simulink model "simulatore"  (R2024a)
settings: Solver=VariableStepAuto  StartTime=0.0  StopTime=0  RelTol=1e-3
values from neighbouring files (symbols this model uses):
  alpharad = (alpha*pi)/180    [cl_alpha.m]
  cd0 = 0.01    [cambio_performance.m]    (also in simulazione_trimmaggio.m; verfica_validazione.m)
  Cl = ext_nl_CLalfa_XLS(:,2)'    [cl_alpha.m]
  deltaT_conv = (T/(n_engine*Tsl) )*(rho0/rhoz)^nt    [simulazione_trimmaggio.m]
  e = 0.9    [simulazione_trimmaggio.m]
  g = 9.8066    [cambio_performance.m]    (also in simulazione_trimmaggio.m; verfica_validazione.m)
  height_des = height_trim+(1000*0.3048)    (= 1219.2)    [simulazione_trimmaggio.m]
  height_trim = h_ft * 0.3048    [cambio_performance.m]    (also in simulazione_trimmaggio.m = 914.4; verfica_validazione.m)
  lambda = -0.0065    [cambio_performance.m]    (also in simulazione_trimmaggio.m; verfica_validazione.m)
  lambdaD = (wing_span^2) / wing_area    (= 8.57002616279)    [cambio_performance.m]    (also in simulazione_trimmaggio.m; verfica_validazione.m)
  MFC = (2144+2122)*0.4535    (= 1934.631)    [simulazione_trimmaggio.m]
  MTOM = 9163    [cambio_performance.m]    (also in simulazione_trimmaggio.m; verfica_validazione.m)
  nt = 1.4236    [simulazione_trimmaggio.m]
  phiT = (8*pi)/180    (= 0.13962634016)    [cambio_performance.m]    (also in simulazione_trimmaggio.m = 0; verfica_validazione.m = 0)
  R = 287.05    [cambio_performance.m]    (also in simulazione_trimmaggio.m; verfica_validazione.m)
  rho0 = 1.225    [cambio_performance.m]    (also in simulazione_trimmaggio.m; verfica_validazione.m)
  SFC = 0.44*0.45/(0.45*9.81/1000*3600)    (= 0.0124589421226)    [simulazione_trimmaggio.m]
  T0 = 288.15    [cambio_performance.m]    (also in simulazione_trimmaggio.m; verfica_validazione.m)
  thetaT = alphaT+gammaT    (= 0.0349065850399)    [simulazione_trimmaggio.m]
  Tsl = 18.32*(10^3)    (= 18320)    [simulazione_trimmaggio.m]
  v = Mach * Vs    [cambio_performance.m]    (also in simulazione_trimmaggio.m = Mach*Vs; verfica_validazione.m)
  wing_area = 34.4    [cambio_performance.m]    (also in simulazione_trimmaggio.m; verfica_validazione.m)
undefined symbols (not defined in the file or in its folder): magnitude
settings Model: Creator=lisys  LastModifiedBy=Simone

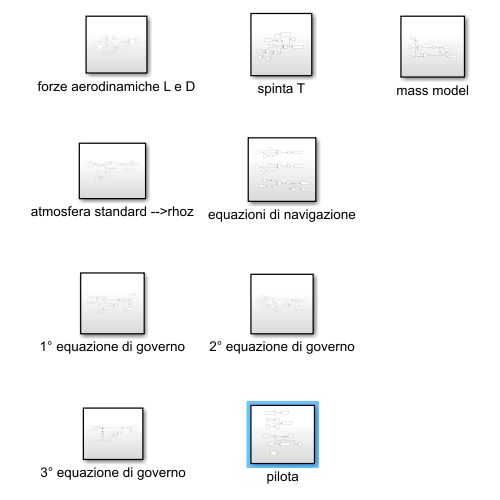
[thumbnail: Simulink's stored preview of the top-level diagram]
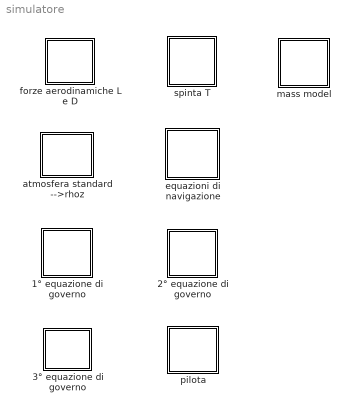
== system simulatore ==
  1° equazione di governo : Subsystem
  2° equazione di governo : Subsystem
  3° equazione di governo : Subsystem
  atmosfera standard -->rhoz : Subsystem
  equazioni di navigazione : Subsystem
  forze aerodinamiche L e D : Subsystem
  mass model : Subsystem
  pilota : Subsystem
  spinta T : Subsystem

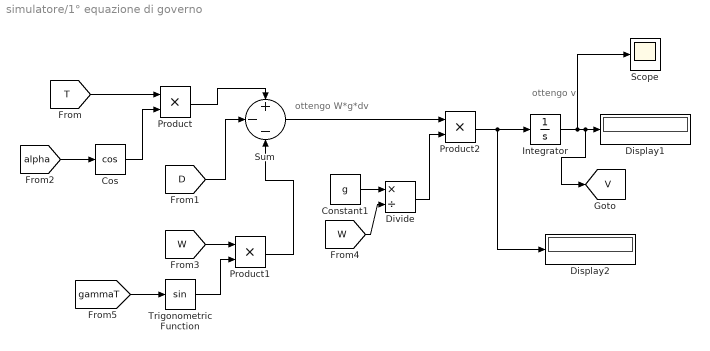
== system simulatore/1° equazione di governo ==
  note: ottengo v
  note: ottengo W*g*dv
  Constant1 : Constant  Value=g
  Cos : Trigonometry  Operator=cos
  Display1 : Display
  Display2 : Display
  Divide : Product  Inputs=*/
  Integrator : Integrator  InitialCondition=v
  Product : Product
  Product1 : Product
  Product2 : Product
  Scope : Scope
  Sum : Sum  Inputs=+--
  Trigonometric Function : Trigonometry
  tag scope: V=global
  wires:
  Integrator/1 -> Scope/1, [V], Display1/1
  [alpha] -> Cos/1
  Trigonometric Function/1 -> Product1/2
  [D] -> Sum/2
  Sum/1 -> Product2/1
  Cos/1 -> Product/2
  Constant1/1 -> Divide/1
  [W] -> Product1/1
  [T] -> Product/1
  Product/1 -> Sum/1
  Divide/1 -> Product2/2
  Product1/1 -> Sum/3
  [W] -> Divide/2
  [gammaT] -> Trigonometric Function/1
  Product2/1 -> Display2/1, Integrator/1

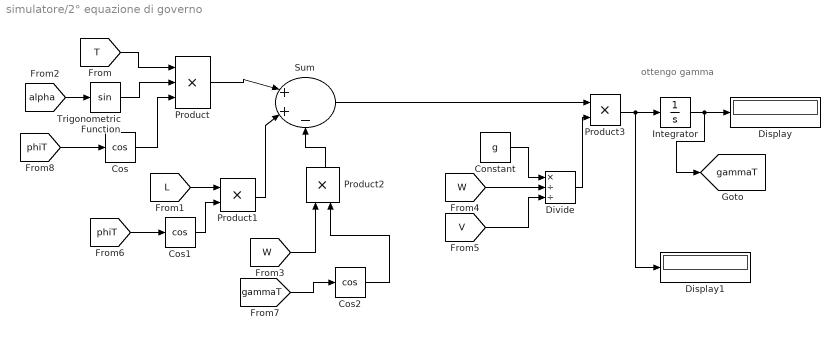
== system simulatore/2° equazione di governo ==
  note: ottengo gamma
  Constant : Constant  Value=g
  Cos : Trigonometry  Operator=cos
  Cos1 : Trigonometry  Operator=cos
  Cos2 : Trigonometry  Operator=cos
  Display : Display
  Display1 : Display
  Divide : Product  Inputs=*//
  Integrator : Integrator
  Product : Product  Inputs=3
  Product1 : Product
  Product2 : Product
  Product3 : Product
  Sum : Sum  Inputs=|++-
  Trigonometric Function : Trigonometry
  tag scope: gammaT=global
  wires:
  Product1/1 -> Sum/2
  [alpha] -> Trigonometric Function/1
  [L] -> Product1/1
  Sum/1 -> Product3/1
  Integrator/1 -> [gammaT], Display/1
  [W] -> Divide/2
  Product2/1 -> Sum/3
  Cos2/1 -> Product2/2
  Cos1/1 -> Product1/2
  Product/1 -> Sum/1
  Divide/1 -> Product3/2
  Cos/1 -> Product/3
  Trigonometric Function/1 -> Product/2
  [W] -> Product2/1
  Product3/1 -> Display1/1, Integrator/1
  [T] -> Product/1
  [phiT] -> Cos1/1
  [gammaT] -> Cos2/1
  [phiT] -> Cos/1
  Constant/1 -> Divide/1
  [V] -> Divide/3

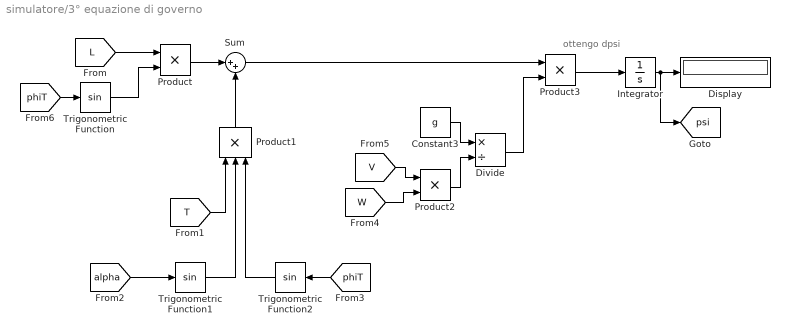
== system simulatore/3° equazione di governo ==
  note: ottengo dpsi
  Constant3 : Constant  Value=g
  Display : Display
  Divide : Product  Inputs=*/
  Integrator : Integrator
  Product : Product
  Product1 : Product  Inputs=3
  Product2 : Product
  Product3 : Product
  Sum : Sum  Inputs=|++
  Trigonometric Function : Trigonometry
  Trigonometric Function1 : Trigonometry
  Trigonometric Function2 : Trigonometry
  tag scope: psi=global
  wires:
  Sum/1 -> Product3/1
  Trigonometric Function/1 -> Product/2
  Product2/1 -> Divide/2
  [alpha] -> Trigonometric Function1/1
  [W] -> Product2/2
  Divide/1 -> Product3/2
  [T] -> Product1/1
  Product3/1 -> Integrator/1
  Trigonometric Function2/1 -> Product1/3
  Integrator/1 -> [psi], Display/1
  Trigonometric Function1/1 -> Product1/2
  Product1/1 -> Sum/2
  Product/1 -> Sum/1
  [L] -> Product/1
  Constant3/1 -> Divide/1
  [V] -> Product2/1
  [phiT] -> Trigonometric Function2/1
  [phiT] -> Trigonometric Function/1

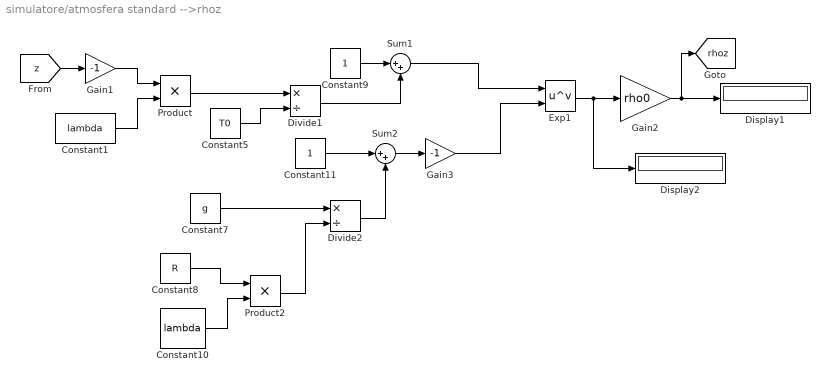
== system simulatore/atmosfera standard -->rhoz ==
  Constant1 : Constant  Value=lambda
  Constant10 : Constant  Value=lambda
  Constant11 : Constant
  Constant5 : Constant  Value=T0
  Constant7 : Constant  Value=g
  Constant8 : Constant  Value=R
  Constant9 : Constant
  Display1 : Display
  Display2 : Display
  Divide1 : Product  Inputs=*/
  Divide2 : Product  Inputs=*/
  Exp1 : Math  Operator=pow
  Gain1 : Gain  Gain=-1
  Gain2 : Gain  Gain=rho0
  Gain3 : Gain  Gain=-1
  Product : Product
  Product2 : Product
  Sum1 : Sum  Inputs=|++
  Sum2 : Sum  Inputs=|++
  tag scope: rhoz=global
  wires:
  Constant10/1 -> Product2/2
  Divide2/1 -> Sum2/2
  Constant5/1 -> Divide1/2
  Exp1/1 -> Display2/1, Gain2/1
  Constant7/1 -> Divide2/1
  Constant9/1 -> Sum1/1
  Constant8/1 -> Product2/1
  Divide1/1 -> Sum1/2
  Product2/1 -> Divide2/2
  Constant11/1 -> Sum2/1
  Sum1/1 -> Exp1/1
  Gain2/1 -> [rhoz], Display1/1
  [z] -> Gain1/1
  Sum2/1 -> Gain3/1
  Gain3/1 -> Exp1/2
  Gain1/1 -> Product/1
  Constant1/1 -> Product/2
  Product/1 -> Divide1/1

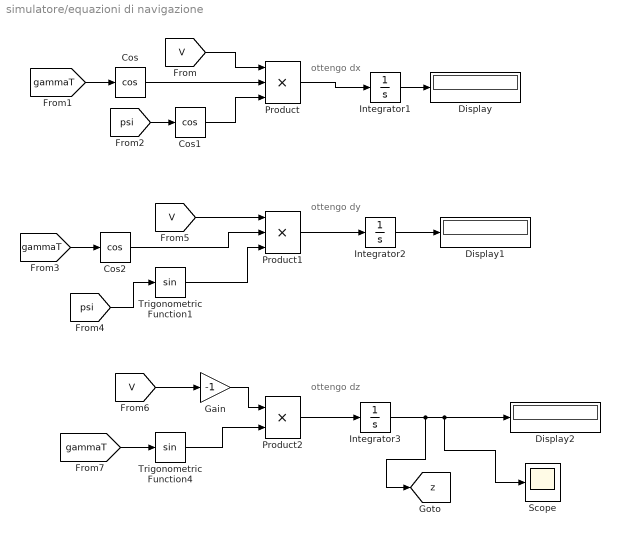
== system simulatore/equazioni di navigazione ==
  note: ottengo dx
  note: ottengo dy
  note: ottengo dz
  Cos : Trigonometry  Operator=cos
  Cos1 : Trigonometry  Operator=cos
  Cos2 : Trigonometry  Operator=cos
  Display : Display
  Display1 : Display
  Display2 : Display
  Gain : Gain  Gain=-1
  Integrator1 : Integrator
  Integrator2 : Integrator
  Integrator3 : Integrator  InitialCondition=-height_trim
  Product : Product  Inputs=3
  Product1 : Product  Inputs=3
  Product2 : Product
  Scope : Scope
  Trigonometric Function1 : Trigonometry
  Trigonometric Function4 : Trigonometry
  tag scope: z=global
  wires:
  Product1/1 -> Integrator2/1
  Product2/1 -> Integrator3/1
  Product/1 -> Integrator1/1
  Trigonometric Function4/1 -> Product2/2
  [V] -> Product/1
  Cos/1 -> Product/2
  Cos1/1 -> Product/3
  [gammaT] -> Cos/1
  [psi] -> Cos1/1
  Integrator1/1 -> Display/1
  Integrator2/1 -> Display1/1
  Cos2/1 -> Product1/2
  Trigonometric Function1/1 -> Product1/3
  [gammaT] -> Cos2/1
  [psi] -> Trigonometric Function1/1
  [V] -> Product1/1
  [V] -> Gain/1
  Gain/1 -> Product2/1
  [gammaT] -> Trigonometric Function4/1
  Integrator3/1 -> [z], Scope/1, Display2/1

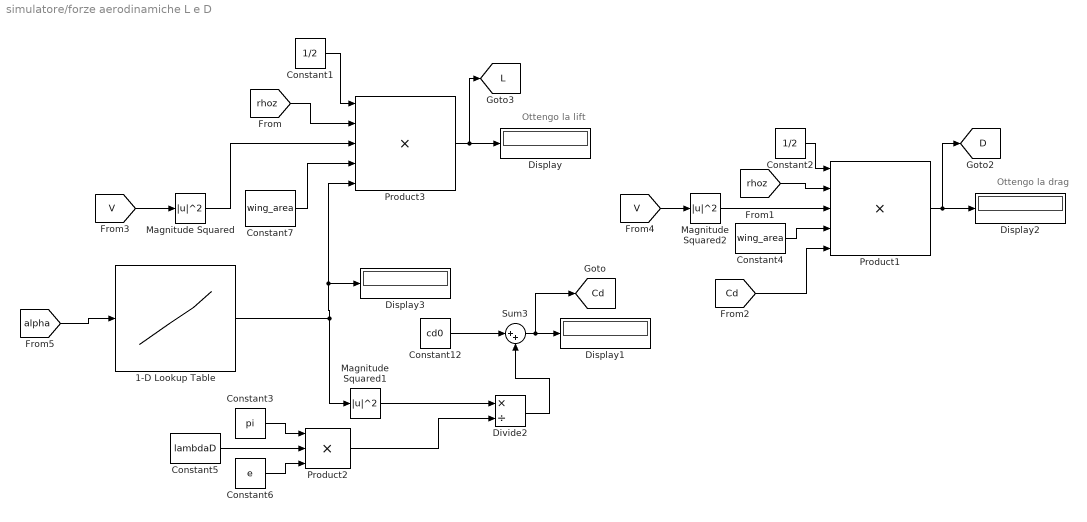
== system simulatore/forze aerodinamiche L e D ==
  note: Ottengo la lift
  note: Ottengo la drag
  1-D Lookup Table : Lookup_n-D  NumberOfTableDimensions=1  BreakpointsForDimension1=alpharad  Table=Cl  InternalRulePriority=Speed  RndMeth=Simplest
  Constant1 : Constant  Value=1/2
  Constant12 : Constant  Value=cd0
  Constant2 : Constant  Value=1/2
  Constant3 : Constant  Value=pi
  Constant4 : Constant  Value=wing_area
  Constant5 : Constant  Value=lambdaD
  Constant6 : Constant  Value=e
  Constant7 : Constant  Value=wing_area
  Display{,1..3} (4 alike) : Display
  Divide2 : Product  Inputs=*/
  Magnitude Squared : Math  Operator=magnitude^2
  Magnitude Squared1 : Math  Operator=magnitude^2
  Magnitude Squared2 : Math  Operator=magnitude^2
  Product1 : Product  Inputs=5
  Product2 : Product  Inputs=3
  Product3 : Product  Inputs=5
  Sum3 : Sum  Inputs=|++
  tag scope: Cd=global, D=global, L=global
  wires:
  Constant1/1 -> Product3/1
  Magnitude Squared1/1 -> Divide2/1
  Product3/1 -> [L], Display/1
  1-D Lookup Table/1 -> Magnitude Squared1/1, Display3/1, Product3/5
  Constant7/1 -> Product3/4
  Constant12/1 -> Sum3/1
  Magnitude Squared/1 -> Product3/3
  Divide2/1 -> Sum3/2
  Sum3/1 -> [Cd], Display1/1
  [rhoz] -> Product3/2
  [rhoz] -> Product1/2
  Magnitude Squared2/1 -> Product1/3
  Constant4/1 -> Product1/4
  Product1/1 -> [D], Display2/1
  Constant2/1 -> Product1/1
  [Cd] -> Product1/5
  [V] -> Magnitude Squared/1
  [V] -> Magnitude Squared2/1
  Constant3/1 -> Product2/1
  Constant5/1 -> Product2/2
  Constant6/1 -> Product2/3
  Product2/1 -> Divide2/2
  [alpha] -> 1-D Lookup Table/1

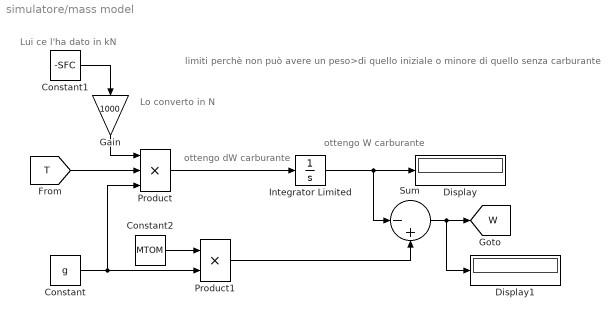
== system simulatore/mass model ==
  note: Lui ce l'ha dato in kN
  note: ottengo dW carburante
  note: limiti perchè non può avere un peso>di quello iniziale o minore di quello senza carburante
  note: ottengo W carburante
  note: Lo converto in N
  Constant : Constant  Value=g
  Constant1 : Constant  Value=-SFC
  Constant2 : Constant  Value=MTOM
  Display : Display
  Display1 : Display
  Gain : Gain  Gain=1000
  Integrator Limited : Integrator  LimitOutput=on  UpperSaturationLimit=MFC*g  LowerSaturationLimit=0
  Product : Product  Inputs=3
  Product1 : Product
  Sum : Sum  Inputs=|-+
  tag scope: W=global
  wires:
  Constant/1 -> Product/3, Product1/2
  Constant1/1 -> Gain/1
  Product/1 -> Integrator Limited/1
  Integrator Limited/1 -> Sum/1, Display/1
  Gain/1 -> Product/1
  Sum/1 -> Display1/1, [W]
  Constant2/1 -> Product1/1
  [T] -> Product/2
  Product1/1 -> Sum/2

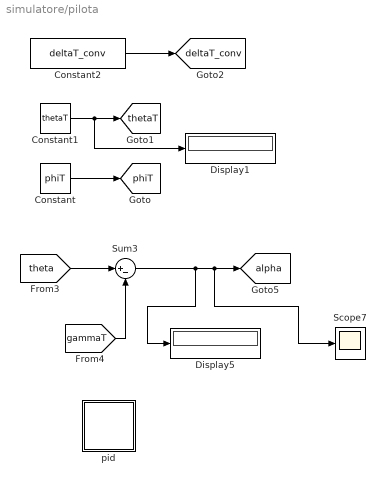
== system simulatore/pilota ==
  Constant : Constant  Value=phiT
  Constant1 : Constant  Value=thetaT
  Constant2 : Constant  Value=deltaT_conv
  Display1 : Display
  Display5 : Display
  Scope7 : Scope
  Sum3 : Sum  Inputs=|+-
  pid : Subsystem
  tag scope: alpha=global, deltaT_conv=global, phiT=global, thetaT=global
  wires:
  Constant/1 -> [phiT]
  Constant2/1 -> [deltaT_conv]
  Constant1/1 -> Display1/1, [thetaT]
  Sum3/1 -> Scope7/1, [alpha], Display5/1
  [theta] -> Sum3/1
  [gammaT] -> Sum3/2

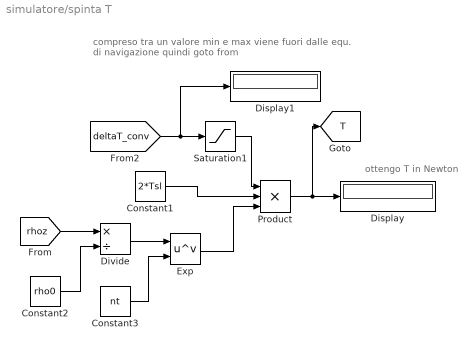
== system simulatore/spinta T ==
  note: compreso tra un valore min e max
      | viene fuori dalle equ. di navigazione quindi goto from
  note: ottengo T in Newton
  Constant1 : Constant  Value=2*Tsl
  Constant2 : Constant  Value=rho0
  Constant3 : Constant  Value=nt
  Display : Display
  Display1 : Display
  Divide : Product  Inputs=*/
  Exp : Math  Operator=pow
  Product : Product  Inputs=3
  Saturation1 : Saturate  UpperLimit=1  LowerLimit=0.015
  tag scope: T=global
  wires:
  Divide/1 -> Exp/1
  Constant2/1 -> Divide/2
  Product/1 -> [T], Display/1
  [rhoz] -> Divide/1
  Constant1/1 -> Product/2
  Constant3/1 -> Exp/2
  Exp/1 -> Product/3
  [deltaT_conv] -> Saturation1/1, Display1/1
  Saturation1/1 -> Product/1

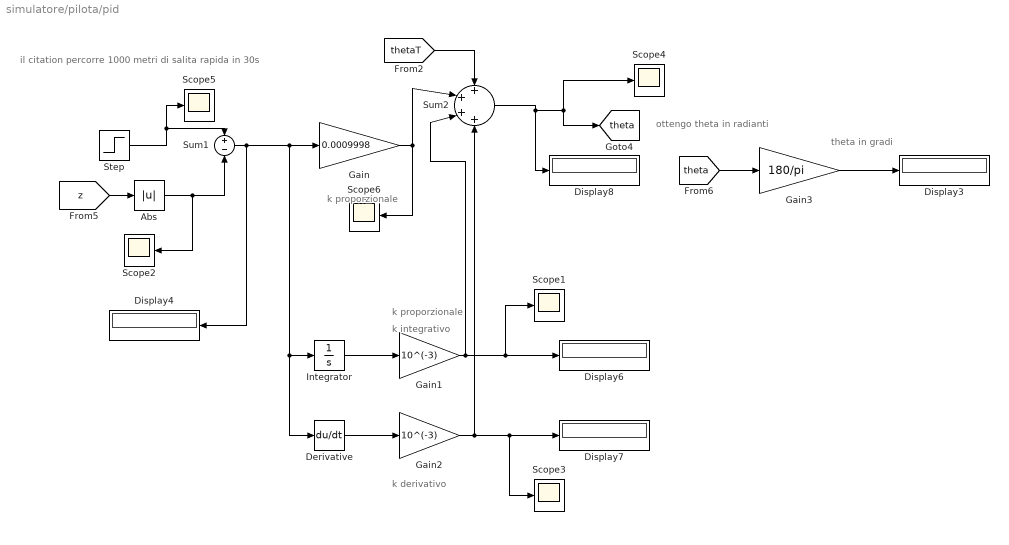
== system simulatore/pilota/pid ==
  note: theta in gradi
  note: il citation percorre 1000 metri di salita rapida in 30s
  note: k proporzionale
  note: k proporzionale
  note: k integrativo
  note: k derivativo
  note: ottengo theta in radianti
  Abs : Abs  SaturateOnIntegerOverflow=off
  Derivative : Derivative
  Display{3..4,6..8} (5 alike) : Display
  Gain : Gain  Gain=0.0009998
  Gain1 : Gain  Gain=10^(-3)
  Gain2 : Gain  Gain=10^(-3)
  Gain3 : Gain  Gain=180/pi
  Integrator : Integrator
  Scope{1..6} (6 alike) : Scope
  Step : Step  Time=30  Before=height_trim  After=height_des  SampleTime=0
  Sum1 : Sum  Inputs=+-
  Sum2 : Sum  Inputs=++++
  tag scope: theta=global
  wires:
  Step/1 -> Scope5/1, Sum1/1
  Gain2/1 -> Scope3/1, Display7/1, Sum2/4
  Integrator/1 -> Gain1/1
  Sum2/1 -> Scope4/1, [theta], Display8/1
  [thetaT] -> Sum2/1
  Gain/1 -> Sum2/2, Scope6/1
  Abs/1 -> Scope2/1, Sum1/2
  Gain1/1 -> Sum2/3, Scope1/1, Display6/1
  Sum1/1 -> Display4/1, Derivative/1, Integrator/1, Gain/1
  Derivative/1 -> Gain2/1
  [z] -> Abs/1
  Gain3/1 -> Display3/1
  [theta] -> Gain3/1
